simulink model "Product"  (R2015b)
settings: Solver=VariableStepAuto  StartTime=0.0  StopTime=10.0  RelTol=1e-3
settings Model: Creator=LUBO  LastModifiedBy=LUBO

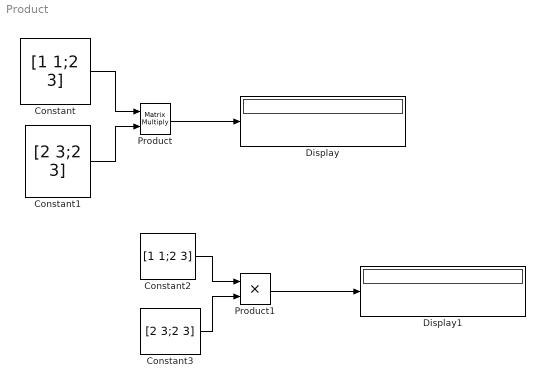
== system Product ==
  Constant : Constant  Value=[1 1;2 3]
  Constant1 : Constant  Value=[2 3;2 3]
  Constant2 : Constant  Value=[1 1;2 3]
  Constant3 : Constant  Value=[2 3;2 3]
  Display : Display
  Display1 : Display
  Product : Product  Multiplication=Matrix(*)
  Product1 : Product
  wires:
  Product/1 -> Display/1
  Constant1/1 -> Product/2
  Constant/1 -> Product/1
  Product1/1 -> Display1/1
  Constant2/1 -> Product1/1
  Constant3/1 -> Product1/2
